simulink model "w1p6"  (R2020b)
settings: Solver=VariableStepAuto  StartTime=0.0  StopTime=10.0  RelTol=1e-3
settings Model: Creator=family  LastModifiedBy=family

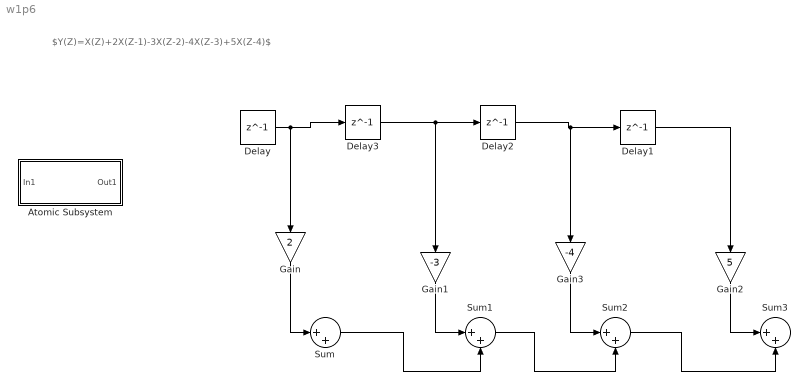
== system w1p6 ==
  note: $Y(Z)=X(Z)+2X(Z-1)-3X(Z-2)-4X(Z-3)+5X(Z-4)$
  Atomic Subsystem : Subsystem  TreatAsAtomicUnit=on
  Delay{,1..3} (4 alike) : Delay  DelayLength=1
  Gain : Gain  Gain=2
  Gain1 : Gain  Gain=-3
  Gain2 : Gain  Gain=5
  Gain3 : Gain  Gain=-4
  Sum{,1..3} (4 alike) : Sum  Inputs=|++
  wires:
  Gain/1 -> Sum/1
  Delay/1 -> Gain/1, Delay3/1
  Delay3/1 -> Gain1/1, Delay2/1
  Delay2/1 -> Gain3/1, Delay1/1
  Sum/1 -> Sum1/2
  Gain1/1 -> Sum1/1
  Gain3/1 -> Sum2/1
  Sum1/1 -> Sum2/2
  Delay1/1 -> Gain2/1
  Gain2/1 -> Sum3/1
  Sum2/1 -> Sum3/2

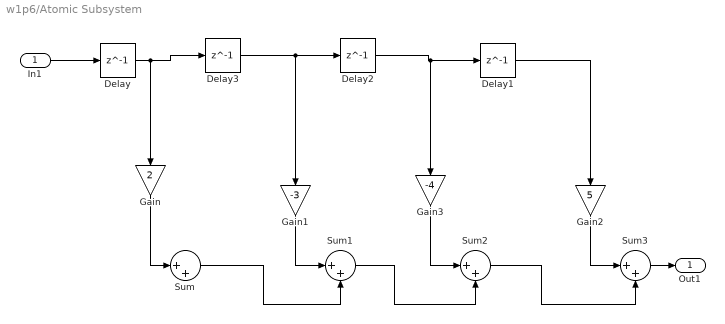
== system w1p6/Atomic Subsystem ==
  In1 : Inport
  Delay{,1..3} (4 alike) : Delay  DelayLength=1
  Gain : Gain  Gain=2
  Gain1 : Gain  Gain=-3
  Gain2 : Gain  Gain=5
  Gain3 : Gain  Gain=-4
  Sum{,1..3} (4 alike) : Sum  Inputs=|++
  Out1 : Outport
  wires:
  Delay3/1 -> Gain1/1, Delay2/1
  Gain2/1 -> Sum3/1
  Sum1/1 -> Sum2/2
  Gain1/1 -> Sum1/1
  Sum2/1 -> Sum3/2
  Delay1/1 -> Gain2/1
  Sum/1 -> Sum1/2
  Delay/1 -> Gain/1, Delay3/1
  Gain3/1 -> Sum2/1
  Gain/1 -> Sum/1
  Delay2/1 -> Gain3/1, Delay1/1
  In1/1 -> Delay/1
  Sum3/1 -> Out1/1
